simulink model "top_level_57_SG_SC_2segs"  (R2025b)
settings: Solver=FixedStepDiscrete  StartTime=0.0  StopTime=50  FixedStep=Ts  RelTol=1e-3
undefined symbols (not defined in the file): DiscIntNeverNeededParam, droop, genTrip, idxa, idxb, idxGenTrip, idxSG_01, idxSMb, mapI_21_3ph, n_genP, n_genQ, n_vRate, n_vRef, noSG, noSM, Pref_lock, rateV, tagI, Ts, wref
libraries: simulink x2, eeGeneralControl x1, eeSinusoidalMeasurementV2 x1, ee_lib_for_power_systems x1
settings Model: SimulationMode=accelerator  ExplicitPartitioning=on  Creator=gdudgeon  LastModifiedBy=gdudgeon
settings DataIOCC: SaveOutput=off  DSMLogging=off  InspectSignalLogs=on  SaveTime=off
settings ModelReferenceCC: UpdateModelReferenceTargets=AssumeUpToDate  ParallelModelReferenceMATLABWorkerInit=Copy Base Workspace

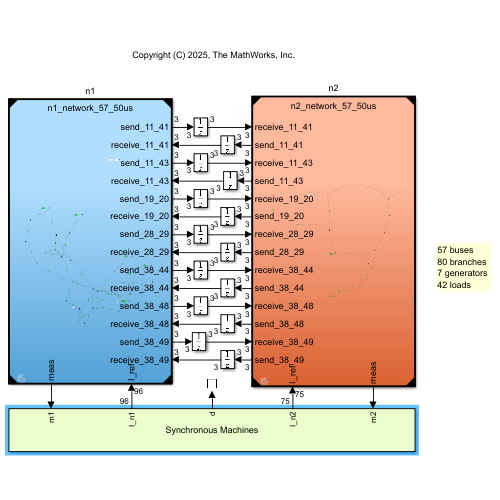
[thumbnail: Simulink's stored preview of the top-level diagram]
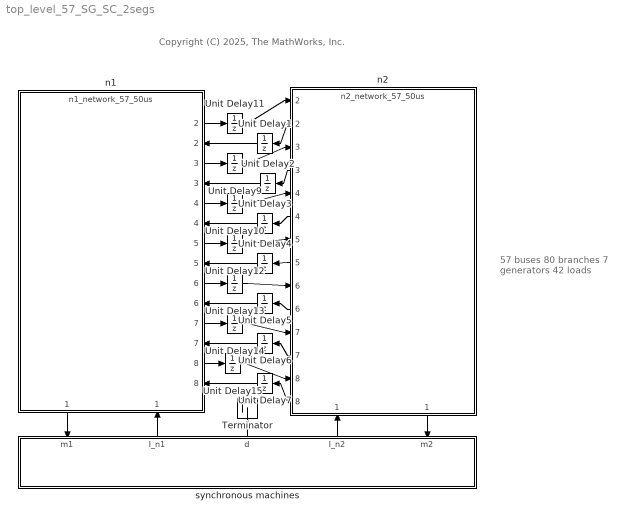
== system top_level_57_SG_SC_2segs ==
  note: Copyright (C) 2025, The MathWorks, Inc.
  note: 57 buses
      | 80 branches
      | 7 generators
      | 42 loads
  Terminator : Terminator
  Unit Delay{1..7,9..15} (14 alike) : UnitDelay  SampleTime=Ts  HasFrameUpgradeWarning=on
  n1 : ModelReference  ModelNameDialog=n1_network_57_50us.slx  ModelReferenceVersion=5.1
      settings: PortSchema="{\"entries\":[{\"content\":{\"sides\":[{\"content\":{},\"type\":\"ConnectorPlacement.EquallySpacedRectSide\",\"uuid\":\"a74df316-1767-4f8a-840d-17e03cd258f4\"},{\"content\":{\"connectorIds\":[\"Out2\",\"In2\",\"Out3\",\"In3\",\"Out4\",\"In4\",\"Out5\",\"In5\",\"Out6\",\"In6\",\"Out7\",\"In7\",\"Out8\",\"In8\"],\"side\":\"RIGHT\"},\"type\":\"ConnectorPlacement.EquallySpacedRectSide\",\"uuid\":\"1b3c021f-69ce-4b13-aefa-cee96e0614ce\"},{\"content\":{\"side\":\"TOP\"},\"type\":\"ConnectorPlacement.EquallySpacedRectSide\",\"uuid\":\"ae15f7f3-c1e2-4a2f-99df-e8d2d0ffd4ae\"},{\"content\":{\"connectorIds\":[\"Out1\",\"In1\"],\"side\":\"BOTTOM\"},\"type\":\"ConnectorPlacement.EquallySpacedRectSide\",\"uuid\":\"649ce0cc-47ac-44c8-b67b-0ed46c10a575\"}]},\"type\":\"ConnectorPlacement.EquallySpacedConnector\",\"uuid\":\"f8de1fa7-a54d-42cb-bb68-f09d9f668e45\"}],\"packageUris\":[\"http://schema.mathworks.com/mf0/Connector/R2020b\"],\"version\":\"1.0\"}"
  n2 : ModelReference  ModelNameDialog=n2_network_57_50us.slx  ModelReferenceVersion=5.1
      settings: PortSchema="{\"entries\":[{\"content\":{\"sides\":[{\"content\":{},\"type\":\"ConnectorPlacement.EquallySpacedRectSide\",\"uuid\":\"a74df316-1767-4f8a-840d-17e03cd258f4\"},{\"content\":{\"connectorIds\":[\"In2\",\"Out2\",\"In3\",\"Out3\",\"In4\",\"Out4\",\"In5\",\"Out5\",\"In6\",\"Out6\",\"In7\",\"Out7\",\"In8\",\"Out8\"],\"side\":\"RIGHT\"},\"type\":\"ConnectorPlacement.EquallySpacedRectSide\",\"uuid\":\"1b3c021f-69ce-4b13-aefa-cee96e0614ce\"},{\"content\":{\"side\":\"TOP\"},\"type\":\"ConnectorPlacement.EquallySpacedRectSide\",\"uuid\":\"ae15f7f3-c1e2-4a2f-99df-e8d2d0ffd4ae\"},{\"content\":{\"connectorIds\":[\"Out1\",\"In1\"],\"side\":\"BOTTOM\"},\"type\":\"ConnectorPlacement.EquallySpacedRectSide\",\"uuid\":\"649ce0cc-47ac-44c8-b67b-0ed46c10a575\"}]},\"type\":\"ConnectorPlacement.EquallySpacedConnector\",\"uuid\":\"f8de1fa7-a54d-42cb-bb68-f09d9f668e45\"}],\"packageUris\":[\"http://schema.mathworks.com/mf0/Connector/R2020b\"],\"version\":\"1.0\"}"
  synchronous machines : Subsystem
      settings: PortSchema="{\"entries\":[{\"content\":{\"sides\":[{\"content\":{},\"type\":\"ConnectorPlacement.EquallySpacedRectSide\",\"uuid\":\"89fdc757-4805-418b-aad8-a8c4d6686521\"},{\"content\":{\"connectorIds\":[\"In1\",\"Out1\",\"Out2\",\"Out3\",\"In2\"],\"side\":\"RIGHT\"},\"type\":\"ConnectorPlacement.EquallySpacedRectSide\",\"uuid\":\"0d4f236b-e24d-4ddb-b314-aac10c72bd50\"},{\"content\":{\"side\":\"TOP\"},\"type\":\"ConnectorPlacement.EquallySpacedRectSide\",\"uuid\":\"7daad4d9-6ba3-46fc-99a4-de53ac5a81f3\"}]},\"type\":\"ConnectorPlacement.EquallySpacedConnector\",\"uuid\":\"9fc17d63-79fb-4d7c-b79f-b0b9b7115830\"}],\"packageUris\":[\"http://schema.mathworks.com/mf0/Connector/R2020b\"],\"version\":\"1.0\"}"
      mask Display: disp('Synchronous Machines')
  wires:
  n1/1 -> synchronous machines/1(m1)
  n2/1 -> synchronous machines/2(m2)
  synchronous machines/2(d) -> Terminator/1
  synchronous machines/1(I_n1) -> n1/1
  synchronous machines/3(I_n2) -> n2/1
  n2/2 -> Unit Delay1/1
  n2/3 -> Unit Delay2/1
  n2/4 -> Unit Delay3/1
  n2/5 -> Unit Delay4/1
  n2/6 -> Unit Delay5/1
  n2/7 -> Unit Delay6/1
  n2/8 -> Unit Delay7/1
  n1/2 -> Unit Delay11/1
  n1/3 -> Unit Delay9/1
  n1/4 -> Unit Delay10/1
  n1/5 -> Unit Delay12/1
  n1/6 -> Unit Delay13/1
  n1/7 -> Unit Delay14/1
  n1/8 -> Unit Delay15/1
  Unit Delay11/1 -> n2/2
  Unit Delay1/1 -> n1/2
  Unit Delay2/1 -> n1/3
  Unit Delay3/1 -> n1/4
  Unit Delay4/1 -> n1/5
  Unit Delay5/1 -> n1/6
  Unit Delay6/1 -> n1/7
  Unit Delay7/1 -> n1/8
  Unit Delay9/1 -> n2/3
  Unit Delay10/1 -> n2/4
  Unit Delay12/1 -> n2/5
  Unit Delay13/1 -> n2/6
  Unit Delay14/1 -> n2/7
  Unit Delay15/1 -> n2/8

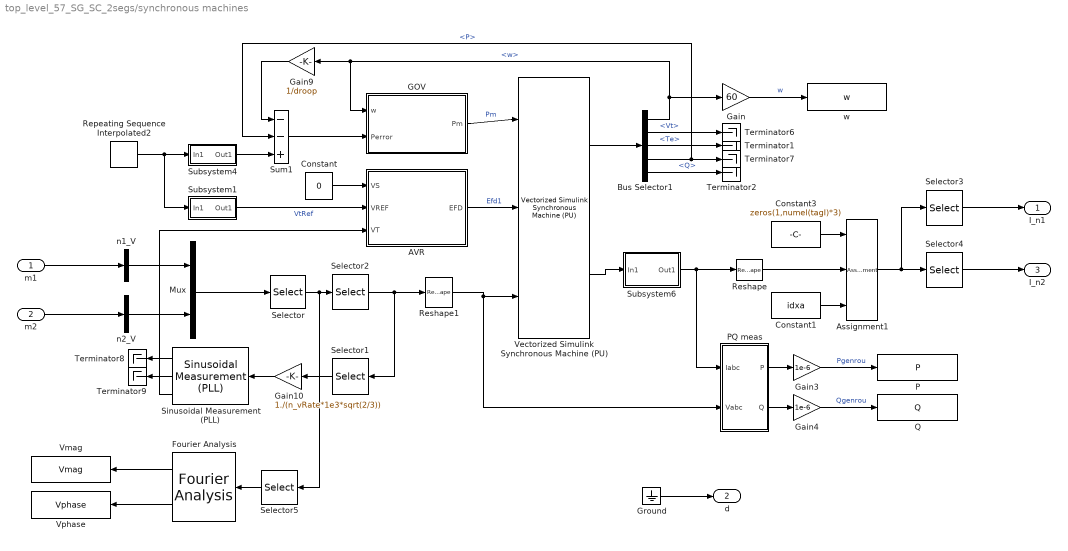
== system top_level_57_SG_SC_2segs/synchronous machines ==
  m1 : Inport  OutDataTypeStr=Bus: n1_slBus3  SampleTime=[5.0000000000000002e-05,0]  BusOutputAsStruct=on
  m2 : Inport  Port=2  OutDataTypeStr=Bus: n2_slBus3  SampleTime=[5.0000000000000002e-05,0]  BusOutputAsStruct=on
  AVR : Subsystem  mask{K=500*ones(1,numel(idxSMb)), TE=0.05*ones(1,numel(idxSMb)), EMIN=0*ones(1,numel(idxSMb)), EMAX=4*ones(1,numel(idxSMb))}
      mask Display: disp('AVR')
  Assignment1 : Assignment  IndexOptions=Index vector (port)  Indices=1  OutputSizes=1
  Bus Selector1 : BusSelector  OutputSignals=w,Vt,Te,P,Q
  Constant : Constant  Value=0  SampleTime=Ts
  Constant1 : Constant  Value=idxa  SampleTime=Ts
  Constant3 : Constant  Value=zeros(1,numel(tagI)*3)  SampleTime=Ts
  Fourier Analysis : eeGeneralControl/Fourier Analysis  f=freq  n=1  M0=1  Ph0=0  BufferSize=8192  Ts=Ts
      settings: LibrarySourceBlock=ee_sl_lib/General Control/Fourier Analysis
  GOV : Subsystem
      mask Display: disp('GOV')
  Gain : Gain  Gain=60
  Gain10 : Gain  Gain=1./(n_vRate*1e3*sqrt(2/3))
  Gain3 : Gain  Gain=1e-6
  Gain4 : Gain  Gain=1e-6
  Gain9 : Gain  Gain=1/droop
  Ground : Ground
  Mux : Mux  Inputs=2
  P : ToWorkspace  VariableName=P  SaveFormat=Timeseries  SampleTime=Ts
  PQ meas : Subsystem  DialogController=POWERSYS.PowerSysDialog
      settings: LibrarySourceBlock=|
      | sps_lib/Sensors and Measurements/Power
      | (3ph, Instantaneous)
  Q : ToWorkspace  VariableName=Q  SaveFormat=Timeseries  SampleTime=Ts
  Repeating Sequence Interpolated2 : simulink/Sources/Repeating Sequence Interpolated  OutValues=[0 0 1 1]  TimeValues=[0 0.2 1 110]  LookUpMeth=Interpolation-Use End Values  tsamp=Ts  OutMin=[]  OutMax=[]  OutDataTypeStr=double  OutputDataTypeScalingMode=double  OutDataType=fixdt(0,8)  OutScaling=2^-10
  Reshape : Reshape
  Reshape1 : Reshape  OutputDimensionality=Customize  OutputDimensions=[3,numel(idxb)]
  Selector : Selector  InputPortWidth=numel(mapI_21_3ph)  IndexOptions=Index vector (dialog)  Indices=mapI_21_3ph  OutputSizes=1
  Selector1 : Selector  InputPortWidth=numel(idxb)*3  IndexOptions=Index vector (dialog)  Indices=1:3:numel(idxb)*3  OutputSizes=1
  Selector2 : Selector  InputPortWidth=numel(tagI)*3  IndexOptions=Index vector (dialog)  Indices=idxa  OutputSizes=1
  Selector3 : Selector  InputPortWidth=numel(tagI)*3  IndexOptions=Index vector (dialog)  Indices=map_tagI2n1_3ph  OutputSizes=1
  Selector4 : Selector  InputPortWidth=numel(tagI)*3  IndexOptions=Index vector (dialog)  Indices=map_tagI2n2_3ph  OutputSizes=1
  Selector5 : Selector  InputPortWidth=57*3  IndexOptions=Index vector (dialog)  Indices=1:3:(57*3)  OutputSizes=1
  Sinusoidal Measurement (PLL) : eeSinusoidalMeasurementV2/Sinusoidal Measurement (PLL)  Ki_PD=1000  Kp_LF=400  Ki_LF=20000  F0=60  Theta0=0  Mag0=0  Ts=Ts
      settings: LibrarySourceBlock=|
      | ee_sl_lib/Measurements/Sinusoidal Measurement
      | (PLL)
  Subsystem1 : Subsystem
  Subsystem4 : Subsystem
  Subsystem6 : Subsystem  mask{tn=idxGenTrip}
      mask prompts: tn "Generator index"
      mask Display: disp('TRIP')
  Sum1 : Sum  Inputs=--+
  Terminator{1..2,6..9} (6 alike) : Terminator
  Vectorized Simulink Synchronous Machine (PU) : ee_lib_for_power_systems/Electromechanical Machines/Vectorized Simulink Synchronous Machine (PU)  Pnom=nomP_SM  Vnom=rateV(idxSMb)*1e3  fnom=60*ones(1,noSM)  NPP=4*ones(1,noSM)  Ra=0.05*ones(1,noSM)  Xl=0.1*ones(1,noSM)  Xd=1.5*ones(1,noSM)  Xq=1.4*ones(1,noSM)  Xdp=0.4*ones(1,noSM)  Xqp=0.5*ones(1,noSM)  Xdpp=0.25*ones(1,noSM)  Xqpp=0.25*ones(1,noSM)  Tdop=5*ones(1,noSM)  Tqop=1.5*ones(1,noSM)  Tdopp=0.6*ones(1,noSM)  Tqopp=0.06*ones(1,noSM)  H=4*ones(1,noSM)  D=zeros(1,noSM)  SatX=SatX  xVec=xVec  no_gens=noSM
      settings: SourceProductName=Support Library for Power Systems
  Vmag : ToWorkspace  VariableName=Vmag  SaveFormat=Timeseries  SampleTime=Ts
  Vphase : ToWorkspace  VariableName=Vphase  SaveFormat=Timeseries  SampleTime=Ts
  n1_V : BusSelector  OutputSignals=V_135kV.Vb_1,V_135kV.Vb_10,V_135kV.Vb_11,V_135kV.Vb_12,V_135kV.Vb_13,V_135kV.Vb_14,V_135kV.Vb_15,V_135kV.Vb_16,V_135kV.Vb_17,V_135kV.Vb_18,V_135kV.Vb_19,V_135kV.Vb_2,V_135kV.Vb_29,V_135kV.Vb_3,V_135kV.Vb_4,V_135kV.Vb_44,V_135kV.Vb_45,V_135kV.Vb_46,V_135kV.Vb_47,V_135kV.Vb_48,V_135kV.Vb_49,V_135kV.Vb_5,V_135kV.Vb_50,V_135kV.Vb_51,V_135kV.Vb_52,V_135kV.Vb_53,V_135kV.Vb_54,V_135kV.Vb_55,V_135kV.Vb_6,V_135kV.Vb_7,V_135kV.Vb_8,V_135kV.Vb_9  OutputAsBus=on
  n2_V : BusSelector  OutputSignals=V_135kV.Vb_20,V_135kV.Vb_21,V_135kV.Vb_22,V_135kV.Vb_23,V_135kV.Vb_24,V_135kV.Vb_25,V_135kV.Vb_26,V_135kV.Vb_27,V_135kV.Vb_28,V_135kV.Vb_30,V_135kV.Vb_31,V_135kV.Vb_32,V_135kV.Vb_33,V_135kV.Vb_34,V_135kV.Vb_35,V_135kV.Vb_36,V_135kV.Vb_37,V_135kV.Vb_38,V_135kV.Vb_39,V_135kV.Vb_40,V_135kV.Vb_41,V_135kV.Vb_42,V_135kV.Vb_43,V_135kV.Vb_56,V_135kV.Vb_57  OutputAsBus=on
  w : ToWorkspace  VariableName=w  SaveFormat=Timeseries  SampleTime=Ts
  I_n1 : Outport  OutDataTypeStr=double  PortDimensions=96  SampleTime=[5.0000000000000002e-05,0]
  d : Outport  Port=2  OutDataTypeStr=double  PortDimensions=1  SampleTime=[5.0000000000000002e-05,0]
  I_n2 : Outport  Port=3  OutDataTypeStr=double  PortDimensions=75  SampleTime=[5.0000000000000002e-05,0]
  wires:
  Bus Selector1/3 -> Terminator1/1  "<Te>"
  Reshape1/1 -> Vectorized Simulink Synchronous Machine (PU)/3, PQ meas/2(Vabc)
  Selector2/1 -> Reshape1/1, Selector1/1
  Gain3/1 -> P/1  "Pgenrou"
  Sinusoidal Measurement (PLL)/2 -> Terminator9/1
  Subsystem6/1(Out1) -> PQ meas/1(Iabc), Reshape/1
  Ground/1 -> d/1
  Vectorized Simulink Synchronous Machine (PU)/2 -> Subsystem6/1(In1)
  Gain4/1 -> Q/1  "Qgenrou"
  m1/1 -> n1_V/1
  Bus Selector1/1 -> GOV/1(w), Gain9/1, Gain/1  "<w>"
  n1_V/1 -> Mux/1
  Bus Selector1/2 -> Terminator6/1  "<Vt>"
  Constant3/1 -> Assignment1/1
  Bus Selector1/5 -> Terminator2/1  "<Q>"
  Repeating Sequence Interpolated2/1 -> Subsystem4/1(In1), Subsystem1/1(In1)
  Subsystem1/1(Out1) -> AVR/2(VREF)  "VtRef"
  Selector3/1 -> I_n1/1
  Selector/1 -> Selector2/1, Selector5/1
  GOV/1(Pm) -> Vectorized Simulink Synchronous Machine (PU)/1  "Pm"
  n2_V/1 -> Mux/2
  Reshape/1 -> Assignment1/2
  Sinusoidal Measurement (PLL)/1 -> Terminator8/1
  Vectorized Simulink Synchronous Machine (PU)/1 -> Bus Selector1/1
  Selector5/1 -> Fourier Analysis/1
  Sinusoidal Measurement (PLL)/3 -> AVR/3(VT)
  AVR/1(EFD) -> Vectorized Simulink Synchronous Machine (PU)/2  "Efd1"
  Constant1/1 -> Assignment1/3
  Sum1/1 -> GOV/2(Perror)
  Subsystem4/1(Out1) -> Sum1/3
  Constant/1 -> AVR/1(VS)
  PQ meas/2(Q) -> Gain4/1
  Gain9/1 -> Sum1/1
  Selector4/1 -> I_n2/1
  Assignment1/1 -> Selector4/1, Selector3/1
  m2/1 -> n2_V/1
  Fourier Analysis/1 -> Vmag/1
  Mux/1 -> Selector/1
  Gain10/1 -> Sinusoidal Measurement (PLL)/1
  Gain/1 -> w/1  "w"
  Fourier Analysis/2 -> Vphase/1
  Selector1/1 -> Gain10/1
  PQ meas/1(P) -> Gain3/1
  Bus Selector1/4 -> Terminator7/1, Sum1/2  "<P>"

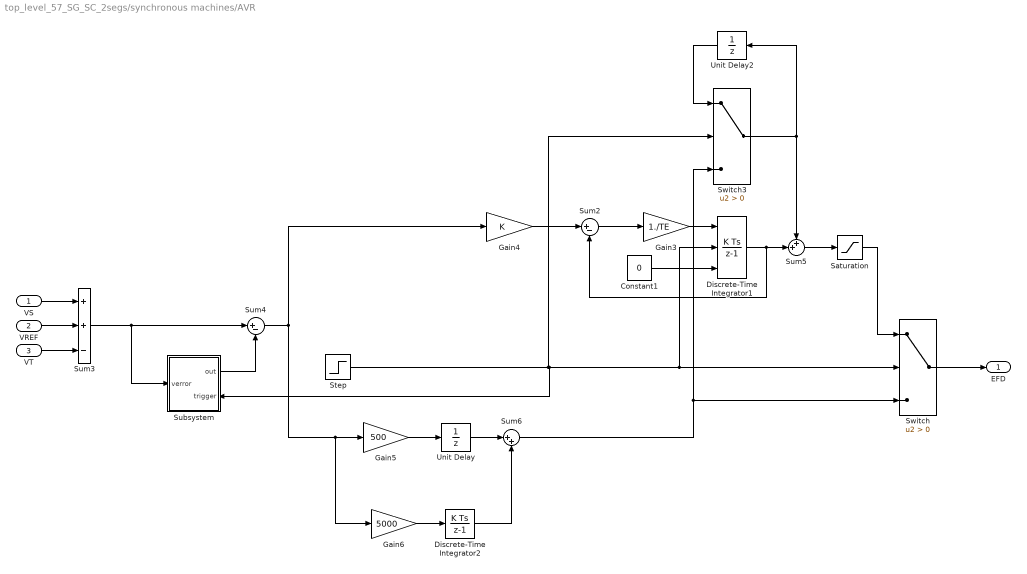
== system top_level_57_SG_SC_2segs/synchronous machines/AVR ==
  VS : Inport
  VREF : Inport  Port=2
  VT : Inport  Port=3
  Constant1 : Constant  Value=0  SampleTime=Ts
  Discrete-Time Integrator1 : DiscreteIntegrator  ExternalReset=rising  InitialConditionSource=external  SampleTime=Ts  UpperSaturationLimit=EMAX  LowerSaturationLimit=EMIN  ICPrevOutput=DiscIntNeverNeededParam  ICPrevScaledInput=DiscIntNeverNeededParam
  Discrete-Time Integrator2 : DiscreteIntegrator  SampleTime=-1  ICPrevOutput=DiscIntNeverNeededParam  ICPrevScaledInput=DiscIntNeverNeededParam
  Gain3 : Gain  Gain=1./TE
  Gain4 : Gain  Gain=K
  Gain5 : Gain  Gain=500
  Gain6 : Gain  Gain=5000
  Saturation : Saturate  UpperLimit=EMAX  LowerLimit=EMIN
  Step : Step  Time=Pref_lock  SampleTime=Ts
  Subsystem : Subsystem
      settings: PortSchema="{\"entries\":[{\"content\":{\"sides\":[{\"content\":{\"connectorIds\":[\"In1\"]},\"type\":\"ConnectorPlacement.EquallySpacedRectSide\",\"uuid\":\"fcea7782-709e-438a-a641-262ec3f31354\"},{\"content\":{\"connectorIds\":[\"Out1\",\"In2\"],\"side\":\"RIGHT\"},\"type\":\"ConnectorPlacement.EquallySpacedRectSide\",\"uuid\":\"9571ea79-f1f3-4aec-b926-22759d29ebce\"},{\"content\":{\"side\":\"TOP\"},\"type\":\"ConnectorPlacement.EquallySpacedRectSide\",\"uuid\":\"bf0a6030-28c1-4408-9c1d-af564ece2abc\"}]},\"type\":\"ConnectorPlacement.EquallySpacedConnector\",\"uuid\":\"5fd903bf-193d-421d-8000-bea997fdfc71\"}],\"packageUris\":[\"http://schema.mathworks.com/mf0/Connector/R2020b\"],\"version\":\"1.0\"}"
  Sum2 : Sum  Inputs=|+-
  Sum3 : Sum  Inputs=++-
  Sum4 : Sum  Inputs=|+-
  Sum5 : Sum  Inputs=++|
  Sum6 : Sum  Inputs=|++
  Switch : Switch  Criteria=u2 > Threshold  SaturateOnIntegerOverflow=off  InputSameDT=off
  Switch3 : Switch  Criteria=u2 > Threshold  SaturateOnIntegerOverflow=off  InputSameDT=off
  Unit Delay : UnitDelay  SampleTime=Ts  HasFrameUpgradeWarning=on
  Unit Delay2 : UnitDelay  SampleTime=Ts  HasFrameUpgradeWarning=on
  EFD : Outport
  wires:
  VS/1 -> Sum3/1
  VREF/1 -> Sum3/2
  VT/1 -> Sum3/3
  Gain4/1 -> Sum2/1
  Sum2/1 -> Gain3/1
  Gain3/1 -> Discrete-Time Integrator1/1
  Switch/1 -> EFD/1
  Sum6/1 -> Switch3/3, Switch/3
  Step/1 -> Discrete-Time Integrator1/2, Switch/2, Subsystem/2(trigger), Switch3/2
  Discrete-Time Integrator1/1 -> Sum2/2, Sum5/2
  Sum5/1 -> Saturation/1
  Switch3/1 -> Unit Delay2/1, Sum5/1
  Unit Delay2/1 -> Switch3/1
  Constant1/1 -> Discrete-Time Integrator1/3
  Gain5/1 -> Unit Delay/1
  Saturation/1 -> Switch/1
  Gain6/1 -> Discrete-Time Integrator2/1
  Discrete-Time Integrator2/1 -> Sum6/2
  Sum4/1 -> Gain4/1, Gain5/1, Gain6/1
  Unit Delay/1 -> Sum6/1
  Subsystem/1(out) -> Sum4/2
  Sum3/1 -> Subsystem/1(verror), Sum4/1

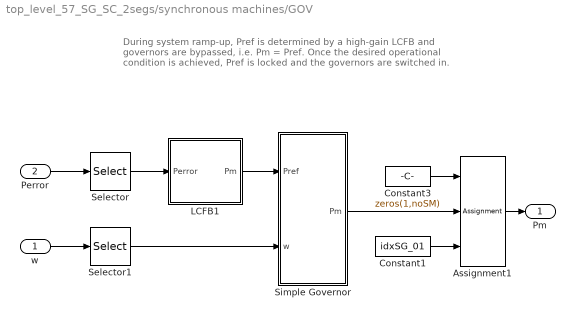
== system top_level_57_SG_SC_2segs/synchronous machines/GOV ==
  note: During system ramp-up, Pref is determined by a high-gain LCFB and governors are bypassed, i.e. Pm = Pref.
      |
      | Once the desired operational condition is achieved, Pref is locked and the governors are switched in.
  w : Inport
  Perror : Inport  Port=2
  Assignment1 : Assignment  IndexOptions=Index vector (port)  Indices=1  OutputSizes=1
  Constant1 : Constant  Value=idxSG_01  SampleTime=Ts
  Constant3 : Constant  Value=zeros(1,noSM)  SampleTime=Ts
  LCFB1 : Subsystem
  Selector : Selector  InputPortWidth=noSM  IndexOptions=Index vector (dialog)  Indices=idxSG_01  OutputSizes=1
  Selector1 : Selector  InputPortWidth=noSM  IndexOptions=Index vector (dialog)  Indices=idxSG_01  OutputSizes=1
  Simple Governor : Subsystem  mask{R=0.2*ones(1,noSG), T1=3*ones(1,noSG), P_MAX=2*ones(1,noSG), P_MIN=0*ones(1,noSG)}
  Pm : Outport
  wires:
  LCFB1/1(Pm) -> Simple Governor/1(Pref)
  Perror/1 -> Selector/1
  w/1 -> Selector1/1
  Simple Governor/1(Pm) -> Assignment1/2
  Constant3/1 -> Assignment1/1
  Constant1/1 -> Assignment1/3
  Assignment1/1 -> Pm/1
  Selector/1 -> LCFB1/1(Perror)
  Selector1/1 -> Simple Governor/2(w)

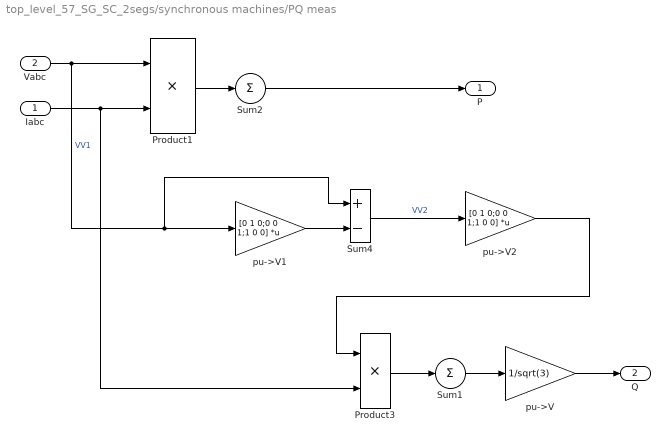
== system top_level_57_SG_SC_2segs/synchronous machines/PQ meas ==
  Iabc : Inport
  Vabc : Inport  Port=2
  Product1 : Product  InputSameDT=on  SaturateOnIntegerOverflow=on  OutDataTypeStr=Inherit: Same as first input
  Product3 : Product  InputSameDT=on  SaturateOnIntegerOverflow=on  OutDataTypeStr=Inherit: Same as first input
  Sum1 : Sum  Inputs=1  CollapseMode=Specified dimension  InputSameDT=on  SaturateOnIntegerOverflow=on  OutDataTypeStr=Inherit: Same as first input
  Sum2 : Sum  Inputs=1  CollapseMode=Specified dimension  InputSameDT=on  SaturateOnIntegerOverflow=on  OutDataTypeStr=Inherit: Same as first input
  Sum4 : Sum  Inputs=+-  InputSameDT=on  SaturateOnIntegerOverflow=on  OutDataTypeStr=Inherit: Same as first input
  pu->V : Gain  Gain=1/sqrt(3)  SaturateOnIntegerOverflow=on  OutDataTypeStr=Inherit: Same as input  ParamDataTypeStr=Inherit: Same as input
  pu->V1 : Gain  Gain=[0 1 0;0 0 1;1 0 0]  Multiplication=Matrix(K*u)  SaturateOnIntegerOverflow=on  OutDataTypeStr=Inherit: Same as input  ParamDataTypeStr=Inherit: Same as input
  pu->V2 : Gain  Gain=[0 1 0;0 0 1;1 0 0]  Multiplication=Matrix(K*u)  SaturateOnIntegerOverflow=on  OutDataTypeStr=Inherit: Same as input  ParamDataTypeStr=Inherit: Same as input
  P : Outport  VectorParamsAs1DForOutWhenUnconnected=off
  Q : Outport  Port=2  VectorParamsAs1DForOutWhenUnconnected=off
  wires:
  pu->V/1 -> Q/1
  Sum1/1 -> pu->V/1
  Product3/1 -> Sum1/1
  Product1/1 -> Sum2/1
  Vabc/1 -> Sum4/1, pu->V1/1, Product1/1  "VV1"
  Iabc/1 -> Product3/2, Product1/2
  Sum2/1 -> P/1
  pu->V1/1 -> Sum4/2
  Sum4/1 -> pu->V2/1  "VV2"
  pu->V2/1 -> Product3/1

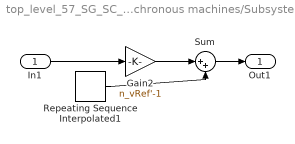
== system top_level_57_SG_SC_2segs/synchronous machines/Subsystem1 ==
  In1 : Inport
  Gain2 : Gain  Gain=n_vRef'-1
  Repeating Sequence Interpolated1 : simulink/Sources/Repeating Sequence Interpolated  OutValues=[0 0 1 1]*1  TimeValues=[0 0.05 0.1 110]  LookUpMeth=Interpolation-Use End Values  tsamp=Ts  OutMin=[]  OutMax=[]  OutDataTypeStr=double  OutputDataTypeScalingMode=double  OutDataType=fixdt(0,8)  OutScaling=2^-10
  Sum : Sum  Inputs=|++
  Out1 : Outport
  wires:
  In1/1 -> Gain2/1
  Sum/1 -> Out1/1
  Repeating Sequence Interpolated1/1 -> Sum/2
  Gain2/1 -> Sum/1

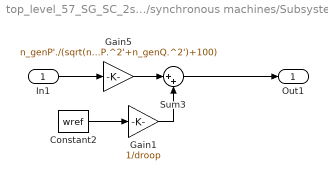
== system top_level_57_SG_SC_2segs/synchronous machines/Subsystem4 ==
  In1 : Inport
  Constant2 : Constant  Value=wref  VectorParams1D=off  SampleTime=Ts
  Gain1 : Gain  Gain=1/droop
  Gain5 : Gain  Gain=n_genP'./(sqrt(n_genP.^2'+n_genQ.^2')+100)
  Sum3 : Sum  Inputs=|++
  Out1 : Outport
  wires:
  Constant2/1 -> Gain1/1
  In1/1 -> Gain5/1
  Gain5/1 -> Sum3/1
  Gain1/1 -> Sum3/2
  Sum3/1 -> Out1/1

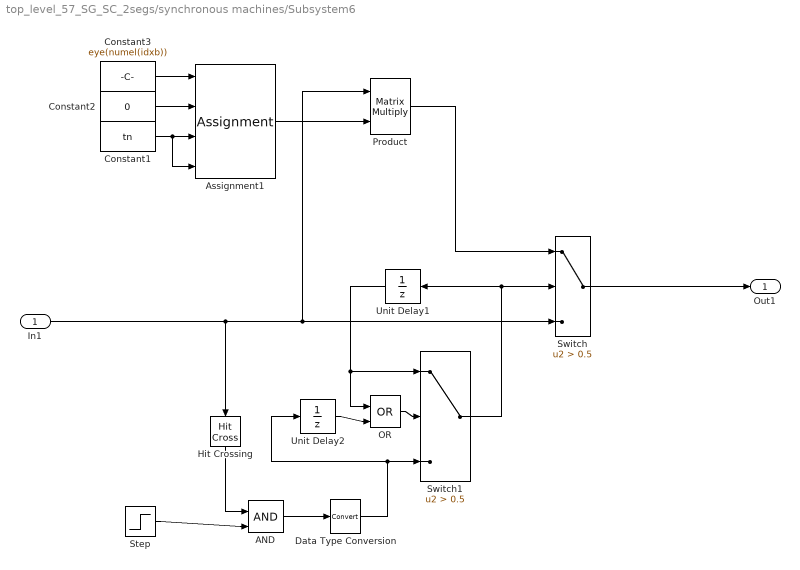
== system top_level_57_SG_SC_2segs/synchronous machines/Subsystem6 ==
  In1 : Inport
  AND : Logic  IconShape=distinctive  AllPortsSameDT=off  OutDataTypeStr=boolean
  Assignment1 : Assignment  NumberOfDimensions=2  IndexOptions=Index vector (port),Index vector (port)  Indices=1,1  OutputSizes=1,1
  Constant1 : Constant  Value=tn  SampleTime=Ts
  Constant2 : Constant  Value=0  SampleTime=Ts
  Constant3 : Constant  Value=eye(numel(idxb))  VectorParams1D=off  SampleTime=Ts
  Data Type Conversion : DataTypeConversion  SaturateOnIntegerOverflow=off  RndMeth=Floor
  Hit Crossing : HitCross
  OR : Logic  Operator=OR  IconShape=distinctive  AllPortsSameDT=off  OutDataTypeStr=boolean
  Product : Product  Multiplication=Matrix(*)
  Step : Step  Time=genTrip  SampleTime=Ts
  Switch : Switch  Criteria=u2 > Threshold  Threshold=0.5  SaturateOnIntegerOverflow=off  InputSameDT=off
  Switch1 : Switch  Criteria=u2 > Threshold  Threshold=0.5  SaturateOnIntegerOverflow=off  InputSameDT=off
  Unit Delay1 : UnitDelay  SampleTime=-1  HasFrameUpgradeWarning=on
  Unit Delay2 : UnitDelay  SampleTime=-1  HasFrameUpgradeWarning=on
  Out1 : Outport
  wires:
  Assignment1/1 -> Product/2
  Constant2/1 -> Assignment1/2
  Constant3/1 -> Assignment1/1
  Constant1/1 -> Assignment1/3, Assignment1/4
  In1/1 -> Switch/3, Product/1, Hit Crossing/1
  Unit Delay2/1 -> OR/2
  AND/1 -> Data Type Conversion/1
  Switch/1 -> Out1/1
  Hit Crossing/1 -> AND/1
  Product/1 -> Switch/1
  OR/1 -> Switch1/2
  Unit Delay1/1 -> Switch1/1, OR/1
  Data Type Conversion/1 -> Switch1/3, Unit Delay2/1
  Switch1/1 -> Switch/2, Unit Delay1/1
  Step/1 -> AND/2

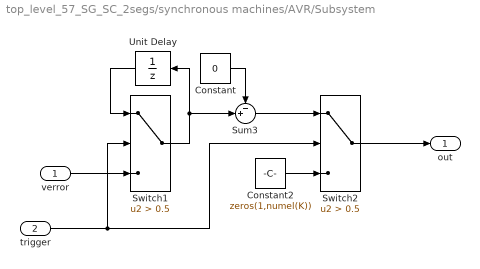
== system top_level_57_SG_SC_2segs/synchronous machines/AVR/Subsystem ==
  verror : Inport
  trigger : Inport  Port=2
  Constant : Constant  Value=0  SampleTime=Ts
  Constant2 : Constant  Value=zeros(1,numel(K))  SampleTime=Ts
  Sum3 : Sum  Inputs=-+|
  Switch1 : Switch  Criteria=u2 > Threshold  Threshold=0.5  SaturateOnIntegerOverflow=off  InputSameDT=off
  Switch2 : Switch  Criteria=u2 > Threshold  Threshold=0.5  SaturateOnIntegerOverflow=off  InputSameDT=off
  Unit Delay : UnitDelay  SampleTime=Ts  HasFrameUpgradeWarning=on
  out : Outport
  wires:
  verror/1 -> Switch1/3
  Switch1/1 -> Sum3/2, Unit Delay/1
  Constant2/1 -> Switch2/3
  trigger/1 -> Switch2/2, Switch1/2
  Unit Delay/1 -> Switch1/1
  Sum3/1 -> Switch2/1
  Switch2/1 -> out/1
  Constant/1 -> Sum3/1

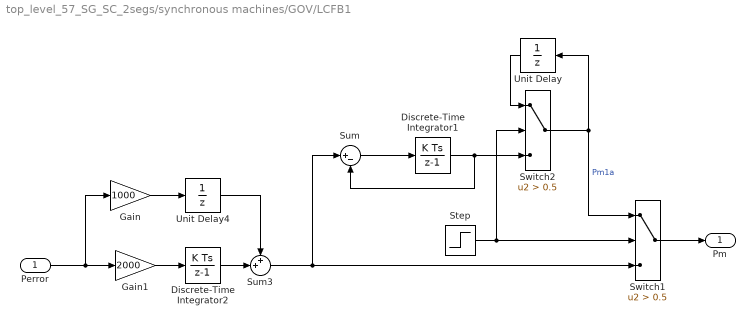
== system top_level_57_SG_SC_2segs/synchronous machines/GOV/LCFB1 ==
  Perror : Inport
  Discrete-Time Integrator1 : DiscreteIntegrator  gainval=10  SampleTime=Ts  LowerSaturationLimit=0  ICPrevOutput=DiscIntNeverNeededParam  ICPrevScaledInput=DiscIntNeverNeededParam
  Discrete-Time Integrator2 : DiscreteIntegrator  gainval=1  SampleTime=Ts  LimitOutput=on  LowerSaturationLimit=0  ICPrevOutput=DiscIntNeverNeededParam  ICPrevScaledInput=DiscIntNeverNeededParam
  Gain : Gain  Gain=1000
  Gain1 : Gain  Gain=2000
  Step : Step  Time=Pref_lock  SampleTime=Ts
  Sum : Sum  Inputs=|+-
  Sum3 : Sum  Inputs=++|
  Switch1 : Switch  Criteria=u2 > Threshold  Threshold=0.5  SaturateOnIntegerOverflow=off  InputSameDT=off
  Switch2 : Switch  Criteria=u2 > Threshold  Threshold=0.5  SaturateOnIntegerOverflow=off  InputSameDT=off
  Unit Delay : UnitDelay  SampleTime=Ts  HasFrameUpgradeWarning=on
  Unit Delay4 : UnitDelay  SampleTime=Ts  HasFrameUpgradeWarning=on
  Pm : Outport
  wires:
  Perror/1 -> Gain/1, Gain1/1
  Unit Delay4/1 -> Sum3/1
  Discrete-Time Integrator2/1 -> Sum3/2
  Switch1/1 -> Pm/1
  Step/1 -> Switch2/2, Switch1/2
  Gain/1 -> Unit Delay4/1
  Gain1/1 -> Discrete-Time Integrator2/1
  Discrete-Time Integrator1/1 -> Switch2/3, Sum/2
  Sum/1 -> Discrete-Time Integrator1/1
  Sum3/1 -> Switch1/3, Sum/1
  Switch2/1 -> Switch1/1, Unit Delay/1  "Pm1a"
  Unit Delay/1 -> Switch2/1

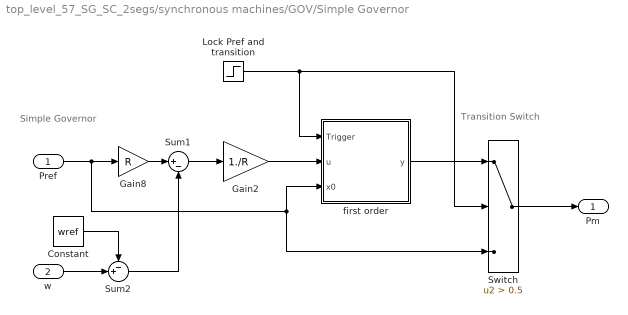
== system top_level_57_SG_SC_2segs/synchronous machines/GOV/Simple Governor ==
  note: Transition Switch
  note: Simple Governor
  Pref : Inport
  w : Inport  Port=2
  Constant : Constant  Value=wref  SampleTime=Ts
  Gain2 : Gain  Gain=1./R
  Gain8 : Gain  Gain=R
  Lock Pref and transition : Step  Time=Pref_lock  SampleTime=Ts
  Sum1 : Sum  Inputs=|+-
  Sum2 : Sum  Inputs=-+|
  Switch : Switch  Criteria=u2 > Threshold  Threshold=0.5  SaturateOnIntegerOverflow=off  InputSameDT=off
  first order : Subsystem
      mask Display: fprintf('1\n------------\n1 + T1s');
  Pm : Outport
  wires:
  Sum1/1 -> Gain2/1
  Pref/1 -> Switch/3, first order/3(x0), Gain8/1
  Switch/1 -> Pm/1
  Lock Pref and transition/1 -> first order/1(Trigger), Switch/2
  first order/1(y) -> Switch/1
  Constant/1 -> Sum2/1
  Sum2/1 -> Sum1/2
  Gain8/1 -> Sum1/1
  Gain2/1 -> first order/2(u)
  w/1 -> Sum2/2

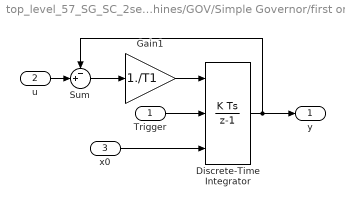
== system top_level_57_SG_SC_2segs/synchronous machines/GOV/Simple Governor/first order ==
  Trigger : Inport
  u : Inport  Port=2
  x0 : Inport  Port=3
  Discrete-Time Integrator : DiscreteIntegrator  ExternalReset=rising  InitialConditionSource=external  SampleTime=Ts  LimitOutput=on  UpperSaturationLimit=P_MAX  LowerSaturationLimit=P_MIN  ICPrevOutput=DiscIntNeverNeededParam  ICPrevScaledInput=DiscIntNeverNeededParam
  Gain1 : Gain  Gain=1./T1
  Sum : Sum  Inputs=-+|
  y : Outport
  wires:
  Trigger/1 -> Discrete-Time Integrator/2
  u/1 -> Sum/2
  Sum/1 -> Gain1/1
  x0/1 -> Discrete-Time Integrator/3
  Discrete-Time Integrator/1 -> y/1, Sum/1
  Gain1/1 -> Discrete-Time Integrator/1
